simulink model "Ueberholmanoever_david"  (R2018a)
settings: Solver=ode1  StartTime=0.0  StopTime=inf  FixedStep=1/10  RelTol=1e-3  EnableMultiTasking=on
undefined symbols (not defined in the file): finding, gray, Lane, PiCar_library, Rec, SDTV
libraries: simulink x15, visiontextngfix x2, visiontransforms x2, visionconversions x1, visionanalysis x1, visionstatistics x1, embdlinuxlib x1
(part 1 of 2)
settings Model: SimulationMode=external  Creator=raspberry  LastModifiedBy=dave
settings SolverCC: PositivePriorityOrder=on
settings OptimizationCC: PassReuseOutputArgsAs=Individual arguments  MaxStackSize=64
settings DebuggingCC: ParameterTunabilityLossMsg=error
settings HardwareCC: ProdBitPerPointer=32  ProdBitPerSizeT=32  ProdBitPerPtrDiffT=32  ProdLargestAtomicInteger=Long  ProdLargestAtomicFloat=Double  ProdWordSize=32  ProdHWDeviceType=ARM Compatible->ARM Cortex
settings RTWCC: SystemTargetFile=ert.tlc  HardwareBoard=Raspberry Pi  TLCOptions="-aInlineSetEventsForThisBaseRateFcn=TLC_FALSE -aSuppressMultiTaskScheduler=TLC_FALSE  -aRateBasedStepFcn=0"  TemplateMakefile=ert_default_tmf  Toolchain=GNU GCC Raspberry Pi
settings RTWCC: CustomTerminator=|
  | /* Send ALL_LED_OFF Signal to all PWM driver chip address
  | See PCA9685 user manual, section 7.3.4
  | Set Chip in sleep mode, section 7.3.1
  | Reset the PWM ON/OFF states for all LEDs */
  | 
  | int fd;
  | 
  | fd = wiringPiI2CSetup(0x70);
  | wiringPiI2CWriteReg8(fd, 0x00, 0x11); // sleep mode
  | wiringPiI2CWriteReg8(fd, 0xFD, 0x10); // all LED off
  | wiringPiI2CWriteReg8(fd, 0xFC, 0x00);
  | wiringPiI2CWriteReg8(fd, 0xFB, 0x00);
  | wiringPiI2CWriteReg8(fd, 0xFA, 0x00);
settings CodeAppCC: ForceParamTrailComments=on  IgnoreCustomStorageClasses=off  OperatorAnnotations=on  SimulinkDataObjDesc=on  SFDataObjDesc=on  MATLABFcnDesc=on  InsertBlockDesc=on  StateflowObjectComments=on  MATLABSourceComments=on
settings ERTTargetCC: SupportVariableSizeSignals=on  ExtMode=on  ExtModeMexArgs='192.168.43.133' 0 17725

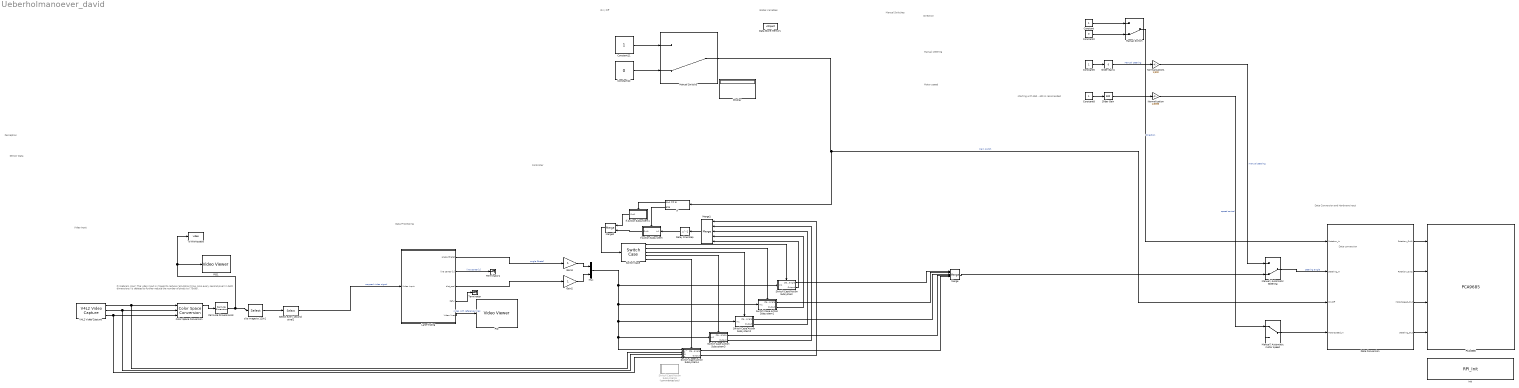
== system Ueberholmanoever_david ==
  note: Manual steering
  note: Sensor Data
  note: Data conversion
  note: Manual Switches
  note: Controller
  note: starting with 350 - 400 is recomended
  note: Data Processing
  note: Data Conversion and Hardware Input
  note: Perception
  note: Pi Webcam Input:
      | The video input is clipped to reduce calculation time. Also every second pixel (in both dimensions) is deleted to further reduce the number of pixels
      | to (75x80).
  note: Direction
  note: Motor speed
  note: Video Input
  note: On / Off
  note: Global Variables
  Color Space Conversion : visionconversions/Color Space  Conversion  conversion=Obsolete  conversionActive=R'G'B' to Y'CbCr  wp_str=D65  rec=Rec. 601 (SDTV)  sys=1125/60/2:1  imagePorts=Separate color signals
      settings: SourceProductName=Computer Vision System Toolbox
  Constant{,5,8,11} (4 alike) : Constant
  Constant12 : Constant  Value=0
  Constant2 : Constant  Value=0
  Data Conversion : Subsystem  AncestorBlock=PiCar_library/Verarbeitung und Datenkonvertierung
  Data Store Memory : DataStoreMemory  DataStoreName=vObject  ReadBeforeWriteMsg=warning  WriteAfterWriteMsg=warning  WriteAfterReadMsg=warning  ShowAdditionalParam=off
  Delay One Step : Delay  DelayLength=1  InitialCondition=1
  Display : Display
  Gain2 : Gain
  Gain3 : Gain
  If : If  IfExpression=u1 == 0
  If Action Subsystem : Subsystem  TreatAsAtomicUnit=on
  If Action Subsystem1 : Subsystem  TreatAsAtomicUnit=on
  Init : S-Function  Priority=1  InitFcn=try, set_param(gcb,'FunctionName','RPI_Init'), end  FunctionName=RPI_Init  SFunctionModules=RPI_Init_wrapper  SFunctionDeploymentMode=off  EnableBusSupport=off  mask(S-Function Builder){}
      mask help: Simulink:masks:SFunctionBuilder_MD
      mask init:
      | val = [[.9  0.75 0.75 1 1 .9 .9 1]',[1 1 0.75 0.75 .9 .9 1 .9]'];try , sys = get_param(gcb,'SfunBuilderFcnName');if isempty(sys), sys = get_param(gcb,'FunctionName'); end,catch, sys = get_param(gcb,'FunctionName'); end
      settings: CopyFcn=set_param(gcbh,'LinkStatus','none')  PreSaveFcn=try, set_param(gcb,'FunctionName','RPI_Init'), end  OpenFcn=sfunctionwizard(gcbh)
      mask Display:
      | plot(val(:,1),val(:,2))
      | disp(sys)
  Lane-finding : Subsystem  AncestorBlock=PiCar_library/Lane-finding
  Manual / Automatic Steering : ManualSwitch  CurrentSetting=0
  "Manual / Automatic motor speed " : ManualSwitch
  Manual Switch : ManualSwitch  CurrentSetting=0
  Manual Switch5 : ManualSwitch  CurrentSetting=0
  Merge : Merge  Inputs=6  InitialOutput=0
  Merge1 : Merge  Inputs=5
  Merge2 : Merge
  Mux : Mux  Inputs=2
  Normalization : Gain  Gain=1/3395
  Normalization1 : Gain  Gain=1/300
  PCA6585 : S-Function  InitFcn=try, set_param(gcb,'FunctionName','PCA9685'), end  FunctionName=PCA9685  SFunctionModules=PCA9685_wrapper  SFunctionDeploymentMode=off  EnableBusSupport=off  mask(S-Function Builder){}
      mask help: Simulink:masks:SFunctionBuilder_MD
      mask init: same as Ueberholmanoever_david/Init
      settings: CopyFcn=set_param(gcbh,'LinkStatus','none')  PreSaveFcn=try, set_param(gcb,'FunctionName','PCA9685'), end  OpenFcn=sfunctionwizard(gcbh)
      mask Display: plot(val(:,1),val(:,2)),disp(sys), port_label('input',1,'IN_1'), port_label('input',2,'IN_2'), port_label('input',3,'PWM'), port_label('input',4,'SERVO')
  PID : VideoViewer  colormapValue=gray(256)  FigPos=[6 1073 939 353]
  PID1 : VideoViewer  colormapValue=gray(256)  FigPos=[1 1038 1539.2 765.6]  OpenAtMdlStart=off
  Permute Dimensions3 : PermuteDimensions
  Select every second pixel2 : Selector  NumberOfDimensions=2  InputPortWidth=3  IndexOptions=Select all,Index vector (dialog)  Indices=[1:2:80],[1:2:160]  OutputSizes=1,1
  Slider Gain : simulink/Math Operations/Slider Gain  gain=500  low=0  high=3395
  Slider Gain1 : simulink/Math Operations/Slider Gain  gain=0  low=-300  high=300
  Switch Case : SwitchCase  CaseConditions={5,4,3,2,1}  ShowDefaultCase=off
  Switch Case Action Subsystem : Subsystem  TreatAsAtomicUnit=on
  Switch Case Action Subsystem1 : Subsystem  TreatAsAtomicUnit=on
  Switch Case Action Subsystem2 : Subsystem  TreatAsAtomicUnit=on
  Switch Case Action Subsystem3 : Subsystem  TreatAsAtomicUnit=on
  Switch Case Action Subsystem4 : Subsystem  TreatAsAtomicUnit=on
  Switch Case Action Subsystem5 : Subsystem  Commented=on  TreatAsAtomicUnit=on
  Terminator : Terminator
  Terminator1 : Terminator
  To Workspace : ToWorkspace  VariableName=video  SaveFormat=Timeseries  SampleTime=-1
  V4L2 Video Capture : embdlinuxlib/V4L2 Video Capture  m_devName='/dev/video0'  roi=[0, 0, 640, 480]  imSizeSelection=320x240  imSize=[640, 480]  pixelFormat=RGB  pixelOrder=Planar  sampleTime=1/10  simOutput=Colorbars  blockPlatform=Raspberry Pi
      settings: SourceProductName=Simulink Support Package for Raspberry Pi Hardware  SourceProductBaseCode=RASPPI
  clip image to 120x1 : Selector  NumberOfDimensions=2  InputPortWidth=3  IndexOptions=Index vector (dialog),Index vector (dialog)  Indices=[150:1:210],[1:2:320]  OutputSizes=1,1
  wires:
  Permute Dimensions3/1 -> clip image to 120x1/1, PID1/1, To Workspace/1
  Color Space Conversion/1 -> Permute Dimensions3/1
  V4L2 Video Capture/3 -> Switch Case Action Subsystem4/4(B), Color Space Conversion/3
  Gain2/1 -> Mux/2
  Lane-finding/5(Video lines) -> PID/1  "video with reference lines"
  Normalization1/1 -> Manual / Automatic Steering/1  "manual steering"
  Constant2/1 -> Manual Switch/2
  Data Conversion/4(Steering_Out) -> PCA6585/4
  Slider Gain/1 -> Normalization/1
  V4L2 Video Capture/1 -> Switch Case Action Subsystem4/2(R), Color Space Conversion/1
  Manual Switch/1 -> Data Conversion/1(Rotation_In)  "Direction"
  Lane-finding/1(angle [theta]) -> Gain3/1  "angle [theta]"
  Normalization/1 -> "Manual / Automatic motor speed "/1  "speed control"
  Select every second pixel2/1 -> Lane-finding/1(Video input)  "cropped video signal"
  Lane-finding/4(Ref_I) -> Terminator/1
  Data Conversion/2(Rotation_Out2) -> PCA6585/2
  Manual / Automatic Steering/1 -> Data Conversion/2(Steering_In)  "steering angle"
  Manual Switch5/1 -> If/1, Data Conversion/3(On/Off)  "main switch"
  Data Conversion/1(Rotation_Out1) -> PCA6585/1
  Data Conversion/3(MotorSpeed_Out) -> PCA6585/3
  Lane-finding/2(line center [y]) -> Terminator1/1  "line center [y]"
  Slider Gain1/1 -> Normalization1/1  "Manual steering"
  Constant5/1 -> Slider Gain1/1
  Constant/1 -> Manual Switch/1
  Constant8/1 -> Slider Gain/1
  Gain3/1 -> Mux/1
  clip image to 120x1/1 -> Select every second pixel2/1
  V4L2 Video Capture/2 -> Switch Case Action Subsystem4/3(G), Color Space Conversion/2
  Constant12/1 -> Manual Switch5/2
  Constant11/1 -> Manual Switch5/1
  "Manual / Automatic motor speed "/1 -> Data Conversion/4(MotorSpeed_In)
  Mux/1 -> Switch Case Action Subsystem4/1(In1), Switch Case Action Subsystem3/1(In2), Switch Case Action Subsystem2/1(In1), Switch Case Action Subsystem1/1(In1), Switch Case Action Subsystem/1(In1)
  Lane-finding/3(dist_real) -> Gain2/1
  Switch Case/1 -> Switch Case Action Subsystem/Action
  Switch Case/2 -> Switch Case Action Subsystem1/Action
  Switch Case/3 -> Switch Case Action Subsystem2/Action
  Switch Case/4 -> Switch Case Action Subsystem3/Action
  Switch Case/5 -> Switch Case Action Subsystem4/Action
  Switch Case Action Subsystem/1(steering angle) -> Merge/1
  Switch Case Action Subsystem1/1(steering angle) -> Merge/2
  Switch Case Action Subsystem2/1(steering angle) -> Merge/3
  Switch Case Action Subsystem3/1(steering angle) -> Merge/4
  Switch Case Action Subsystem4/1(steering angle) -> Merge/5
  Merge/1 -> Manual / Automatic Steering/2
  Switch Case Action Subsystem1/2(Output) -> Merge1/4
  Switch Case Action Subsystem2/2(Output) -> Merge1/3
  Switch Case Action Subsystem3/2(Output) -> Merge1/2
  Switch Case Action Subsystem4/2(Output) -> Merge1/1
  Merge1/1 -> Delay One Step/1
  Switch Case Action Subsystem/2(Output) -> Merge1/5
  If/2 -> If Action Subsystem/Action
  Delay One Step/1 -> If Action Subsystem/1(In1)
  If/1 -> If Action Subsystem1/Action
  If Action Subsystem1/1(Out1) -> Merge2/1
  If Action Subsystem/1(Out1) -> Merge2/2
  Merge2/1 -> Switch Case/1

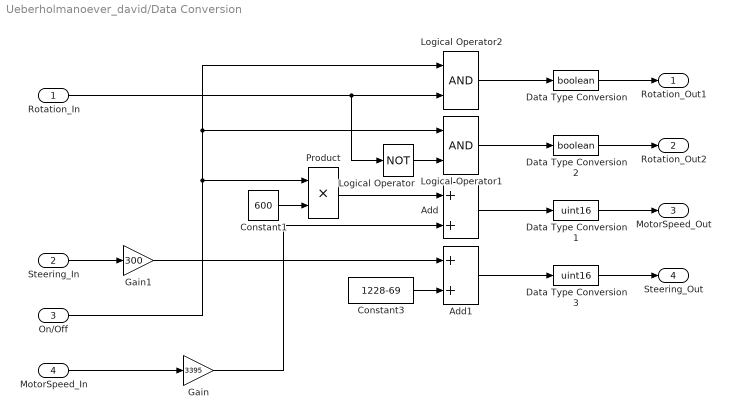
== system Ueberholmanoever_david/Data Conversion ==
  Rotation_In : Inport
  Steering_In : Inport  Port=2
  On/Off : Inport  Port=3
  MotorSpeed_In : Inport  Port=4
  Add : Sum
  Add1 : Sum
  Constant1 : Constant  Value=600
  Constant3 : Constant  Value=1228-69  OutMin=819  OutMax=1638
  Data Type Conversion : DataTypeConversion  OutDataTypeStr=boolean
  Data Type Conversion1 : DataTypeConversion  OutDataTypeStr=uint16
  Data Type Conversion2 : DataTypeConversion  OutDataTypeStr=boolean
  Data Type Conversion3 : DataTypeConversion  OutDataTypeStr=uint16
  Gain : Gain  Gain=3395
  Gain1 : Gain  Gain=300
  Logical Operator : Logic  Operator=NOT  AllPortsSameDT=off  OutDataTypeStr=boolean
  Logical Operator1 : Logic  AllPortsSameDT=off  OutDataTypeStr=boolean
  Logical Operator2 : Logic  AllPortsSameDT=off  OutDataTypeStr=boolean
  Product : Product
  Rotation_Out1 : Outport
  Rotation_Out2 : Outport  Port=2
  MotorSpeed_Out : Outport  Port=3
  Steering_Out : Outport  Port=4
  wires:
  Gain1/1 -> Add1/1
  Gain/1 -> Add/2
  Steering_In/1 -> Gain1/1
  Data Type Conversion/1 -> Rotation_Out1/1
  MotorSpeed_In/1 -> Gain/1
  Data Type Conversion2/1 -> Rotation_Out2/1
  Data Type Conversion3/1 -> Steering_Out/1
  Data Type Conversion1/1 -> MotorSpeed_Out/1
  Product/1 -> Add/1
  Constant1/1 -> Product/2
  Add1/1 -> Data Type Conversion3/1
  Add/1 -> Data Type Conversion1/1
  Rotation_In/1 -> Logical Operator2/2, Logical Operator/1
  Constant3/1 -> Add1/2
  On/Off/1 -> Product/1, Logical Operator2/1, Logical Operator1/1
  Logical Operator/1 -> Logical Operator1/2
  Logical Operator2/1 -> Data Type Conversion/1
  Logical Operator1/1 -> Data Type Conversion2/1

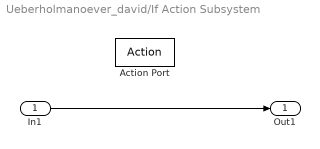
== system Ueberholmanoever_david/If Action Subsystem ==
  In1 : Inport
  Action Port : ActionPort  ActionType=else
  Out1 : Outport
  wires:
  In1/1 -> Out1/1

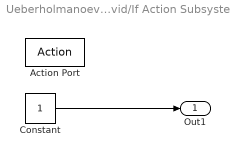
== system Ueberholmanoever_david/If Action Subsystem1 ==
  Action Port : ActionPort  ActionType=then
  Constant : Constant
  Out1 : Outport
  wires:
  Constant/1 -> Out1/1

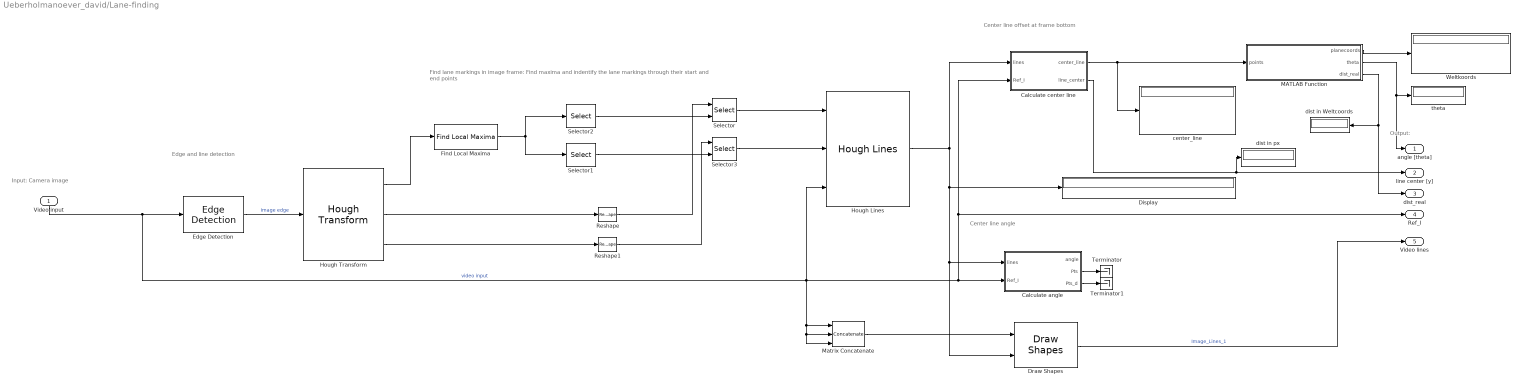
== system Ueberholmanoever_david/Lane-finding ==
  note: Output:
  note: Input: Camera image
  note: Edge and line detection
  note: Find lane markings in image frame:
      | Find maxima and indentify the lane markings through their start and end points
  note: Center line angle
  note: Center line offset at frame bottom
  Video input : Inport
  Calculate angle : MATLAB Function  TreatAsAtomicUnit=on
  Calculate center line : MATLAB Function  TreatAsAtomicUnit=on
  Display : Display
  Draw Shapes : visiontextngfix/Draw Shapes  shape=Lines  fill=off  lineWidth=1  fillClrSource=Specify via dialog  display=User-specified value  intensity=200  color=[0 0 255]  opacity=0.6  viewport=Entire image  antialiasing=off  inType=Obsolete  imagePorts=One multidimensional signal  prodOutputMode=Binary point scaling  prodOutputWordLength=32  prodOutputFracLength=14  memoryMode=Specify word length  memoryWordLength=16  memoryFracLength=14  roundingMode=Floor  overflowMode=off
      settings: SourceProductName=Computer Vision System Toolbox
  Edge Detection : visionanalysis/Edge Detection  method=Sobel  outputType=Binary image  userDefinedThreshold=off  thresholdSource=Input port  threshold=20  thresholdTuning=4  edgeThinning=off  threshold_canny=[0.25 0.60]  autoPercent=70  sigma=1  roundingMode=Floor  overflowMode=off  prodOutputMode=Binary point scaling  prodOutputWordLength=32  prodOutputFracLength=8  prodOutputSlope=2^-8  accumSlope=2^-8  outputSlope=2^-4
      settings: SourceProductName=Computer Vision System Toolbox  SourceProductBaseCode=VP
  Find Local Maxima : visionstatistics/Find Local Maxima  num_peaks=2  nhood_size=[5 7]  src_thresh=Obsolete9b  src_thresh_inuse=Specify via dialog  threshold=10  inputIsHough=off  dt_peak=uint32  isOutVarDim=on  dt_count=uint32
      settings: SourceProductName=Computer Vision System Toolbox  SourceProductBaseCode=VP
  Hough Lines : visiontransforms/Hough Lines  sineCompMethod=Trigonometric function  thetaRes=pi/180  firstCoeffMode=Specify word length  firstCoeffWordLength=16  firstCoeffFracLength=15  prodOutputMode=Binary point scaling  prodOutputWordLength=32  prodOutputFracLength=16  roundingMode=Nearest  overflowMode=on
      settings: SourceProductName=Computer Vision System Toolbox  SourceProductBaseCode=VP
  Hough Transform : visiontransforms/Hough Transform  theta_res=pi/180  rho_res=1  out_theta_rho=on  outdtmode=double  firstCoeffMode=Binary point scaling  firstCoeffWordLength=16  firstCoeffFracLength=14  secondCoeffMode=Binary point scaling  secondCoeffWordLength=32  secondCoeffFracLength=16  outputMode=Binary point scaling  outputWordLength=16  outputFracLength=0  accumMode=Binary point scaling  accumWordLength=32  accumFracLength=20  prodOutputMode=Binary point scaling  prodOutputWordLength=32  prodOutputFracLength=20  memoryMode=Binary point scaling  memoryWordLength=32  memoryFracLength=16  roundingMode=Nearest  overflowMode=on
      settings: SourceProductName=Computer Vision System Toolbox  SourceProductBaseCode=VP
  MATLAB Function : MATLAB Function  TreatAsAtomicUnit=on
  Matrix Concatenate : Concatenate  NumInputs=3  Mode=Multidimensional array  ConcatenateDimension=3
  Reshape : Reshape
  Reshape1 : Reshape
  Selector : Selector  IndexOptions=Index vector (port)  Indices=[1 3]  OutputSizes=1
  Selector1 : Selector  NumberOfDimensions=2  InputPortWidth=3  IndexOptions=Select all,Index vector (dialog)  Indices=[1 3],2  OutputSizes=1,1
  Selector2 : Selector  NumberOfDimensions=2  InputPortWidth=3  IndexOptions=Select all,Index vector (dialog)  Indices=[1 3],1  OutputSizes=1,1
  Selector3 : Selector  IndexOptions=Index vector (port)  Indices=[1 3]  OutputSizes=1
  Terminator : Terminator
  Terminator1 : Terminator
  Weltkoords : Display
  center_line : Display
  dist in Weltcoords : Display
  dist in px : Display
  theta : Display
  angle [theta] : Outport
  line center [y] : Outport  Port=2
  dist_real : Outport  Port=3
  Ref_I : Outport  Port=4
  Video lines : Outport  Port=5
  wires:
  Calculate center line/2(line_center) -> dist in px/1, line center [y]/1
  Hough Lines/1 -> Calculate angle/1(lines), Draw Shapes/2, Display/1, Calculate center line/1(lines)
  Draw Shapes/1 -> Video lines/1  "Image_Lines_1"
  Matrix Concatenate/1 -> Draw Shapes/1
  Reshape1/1 -> Selector3/1
  Selector3/1 -> Hough Lines/2
  Reshape/1 -> Selector/1
  Selector/1 -> Hough Lines/1
  Find Local Maxima/1 -> Selector1/1, Selector2/1
  Selector2/1 -> Selector/2
  Selector1/1 -> Selector3/2
  Hough Transform/1 -> Find Local Maxima/1
  Hough Transform/3 -> Reshape1/1
  Hough Transform/2 -> Reshape/1
  Video input/1 -> Edge Detection/1, Matrix Concatenate/3, Matrix Concatenate/2, Matrix Concatenate/1, Hough Lines/3, Ref_I/1, Calculate center line/2(Ref_I), Calculate angle/2(Ref_I)  "video input"
  Edge Detection/1 -> Hough Transform/1  "Image edge"
  Calculate angle/3(Pts_d) -> Terminator1/1
  Calculate angle/2(Pts) -> Terminator/1
  MATLAB Function/1(planecoords) -> Weltkoords/1
  MATLAB Function/2(theta) -> angle [theta]/1, theta/1
  Calculate center line/1(center_line) -> MATLAB Function/1(points), center_line/1
  MATLAB Function/3(dist_real) -> dist in Weltcoords/1, dist_real/1

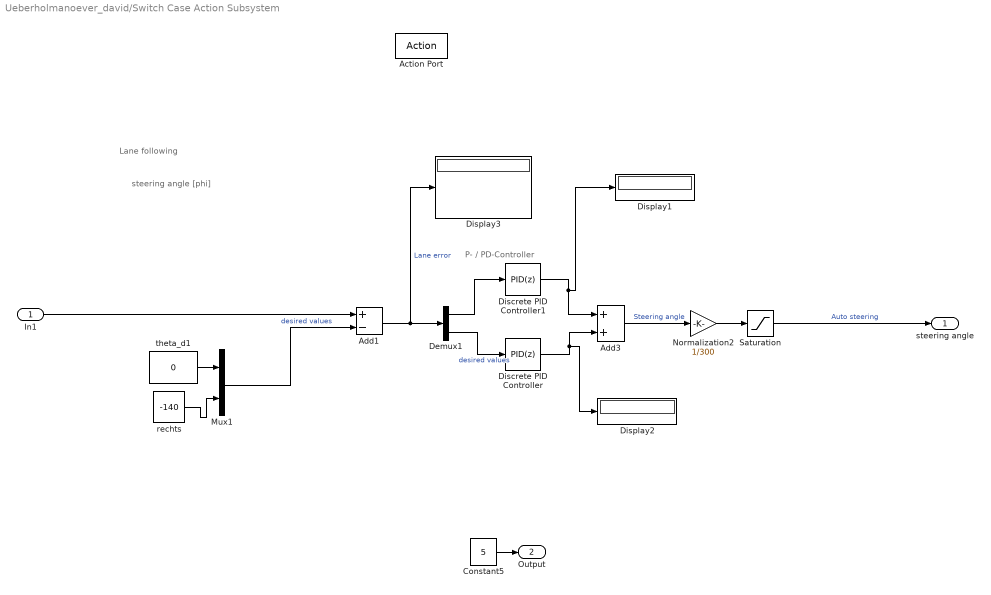
== system Ueberholmanoever_david/Switch Case Action Subsystem ==
  note: steering angle [phi]
  note: P- / PD-Controller
  note: Lane following
  In1 : Inport
  Action Port : ActionPort  ActionType=case
  Add1 : Sum  Inputs=+-
  Add3 : Sum
  Constant5 : Constant  Value=5  OutDataTypeStr=uint8
  Demux1 : Demux  Outputs=2
  Discrete PID Controller : simulink/Continuous/PID Controller  Controller=PID  TimeDomain=Discrete-time  SampleTime=-1  IntegratorMethod=Forward Euler  FilterMethod=Forward Euler  Form=Parallel  UseFilter=on  ControllerParametersSource=internal  P=0.2  I=0  D=0  N=100  InitialConditionSource=internal  InitialConditionForIntegrator=0  InitialConditionForFilter=0  ExternalReset=none  LimitOutput=off  UpperSaturationLimit=inf  LowerSaturationLimit=-inf  LinearizeAsGain=off  AntiWindupMode=none  Kb=1  TrackingMode=off  Kt=1  PParamMin=[]  PParamMax=[]  IParamMin=[]  IParamMax=[]  DParamMin=[]  DParamMax=[]  NParamMin=[]  NParamMax=[]  KbParamMin=[]  KbParamMax=[]  KtParamMin=[]  KtParamMax=[]  POutMin=[]  POutMax=[]  IOutMin=[]  IOutMax=[]  DOutMin=[]  DOutMax=[]  NOutMin=[]  NOutMax=[]  KbOutMin=[]  KbOutMax=[]  KtOutMin=[]  KtOutMax=[]  IntegratorOutMin=[]  IntegratorOutMax=[]  FilterOutMin=[]  FilterOutMax=[]  SumOutMin=[]  SumOutMax=[]  SumI1OutMin=[]  SumI1OutMax=[]  SumI2OutMin=[]  SumI2OutMax=[]  SumI3OutMin=[]  SumI3OutMax=[]  SumDOutMin=[]  SumDOutMax=[]  SaturationOutMin=[]  SaturationOutMax=[]  IntegratorContinuousStateAttributes=''  IntegratorStateMustResolveToSignalObject=off  IntegratorRTWStateStorageClass=Auto  FilterContinuousStateAttributes=''  FilterStateMustResolveToSignalObject=off  FilterRTWStateStorageClass=Auto  DifferentiatorICPrevScaledInput=0  DifferentiatorOutMin=[]  DifferentiatorOutMax=[]  FilterDiffOutCoefMin=[]  FilterDiffOutCoefMax=[]  SumDenOutMin=[]  SumDenOutMax=[]  SumNumOutMin=[]  SumNumOutMax=[]  ReciprocalOutMin=[]  ReciprocalOutMax=[]  DivideOutMin=[]  DivideOutMax=[]  TunerSelectOption=Transfer Function Based (PID Tuner App)
  Discrete PID Controller1 : simulink/Continuous/PID Controller  Controller=PID  TimeDomain=Discrete-time  SampleTime=-1  IntegratorMethod=Forward Euler  FilterMethod=Forward Euler  Form=Parallel  UseFilter=on  ControllerParametersSource=internal  P=6  I=0  D=0  N=100  InitialConditionSource=internal  InitialConditionForIntegrator=0  InitialConditionForFilter=0  ExternalReset=none  LimitOutput=off  UpperSaturationLimit=inf  LowerSaturationLimit=-inf  LinearizeAsGain=off  AntiWindupMode=none  Kb=1  TrackingMode=off  Kt=1  PParamMin=[]  PParamMax=[]  IParamMin=[]  IParamMax=[]  DParamMin=[]  DParamMax=[]  NParamMin=[]  NParamMax=[]  KbParamMin=[]  KbParamMax=[]  KtParamMin=[]  KtParamMax=[]  POutMin=[]  POutMax=[]  IOutMin=[]  IOutMax=[]  DOutMin=[]  DOutMax=[]  NOutMin=[]  NOutMax=[]  KbOutMin=[]  KbOutMax=[]  KtOutMin=[]  KtOutMax=[]  IntegratorOutMin=[]  IntegratorOutMax=[]  FilterOutMin=[]  FilterOutMax=[]  SumOutMin=[]  SumOutMax=[]  SumI1OutMin=[]  SumI1OutMax=[]  SumI2OutMin=[]  SumI2OutMax=[]  SumI3OutMin=[]  SumI3OutMax=[]  SumDOutMin=[]  SumDOutMax=[]  SaturationOutMin=[]  SaturationOutMax=[]  IntegratorContinuousStateAttributes=''  IntegratorStateMustResolveToSignalObject=off  IntegratorRTWStateStorageClass=Auto  FilterContinuousStateAttributes=''  FilterStateMustResolveToSignalObject=off  FilterRTWStateStorageClass=Auto  DifferentiatorICPrevScaledInput=0  DifferentiatorOutMin=[]  DifferentiatorOutMax=[]  FilterDiffOutCoefMin=[]  FilterDiffOutCoefMax=[]  SumDenOutMin=[]  SumDenOutMax=[]  SumNumOutMin=[]  SumNumOutMax=[]  ReciprocalOutMin=[]  ReciprocalOutMax=[]  DivideOutMin=[]  DivideOutMax=[]  TunerSelectOption=Transfer Function Based (PID Tuner App)
  Display1 : Display
  Display2 : Display
  Display3 : Display
  Mux1 : Mux  Inputs=2
  Normalization2 : Gain  Gain=1/300
  Saturation : Saturate  UpperLimit=1  LowerLimit=-1
  rechts : Constant  Value=-140
  theta_d1 : Constant  Value=0
  steering angle : Outport  InitialOutput=[0]
  Output : Outport  Port=2
  wires:
  rechts/1 -> Mux1/2
  Add1/1 -> Display3/1, Demux1/1  "Lane error"
  In1/1 -> Add1/1
  theta_d1/1 -> Mux1/1
  Discrete PID Controller/1 -> Display2/1, Add3/2
  Saturation/1 -> steering angle/1  "Auto steering"
  Normalization2/1 -> Saturation/1
  Discrete PID Controller1/1 -> Display1/1, Add3/1
  Demux1/2 -> Discrete PID Controller/1  "desired values"
  Demux1/1 -> Discrete PID Controller1/1
  Add3/1 -> Normalization2/1  "Steering angle"
  Mux1/1 -> Add1/2  "desired values"
  Constant5/1 -> Output/1

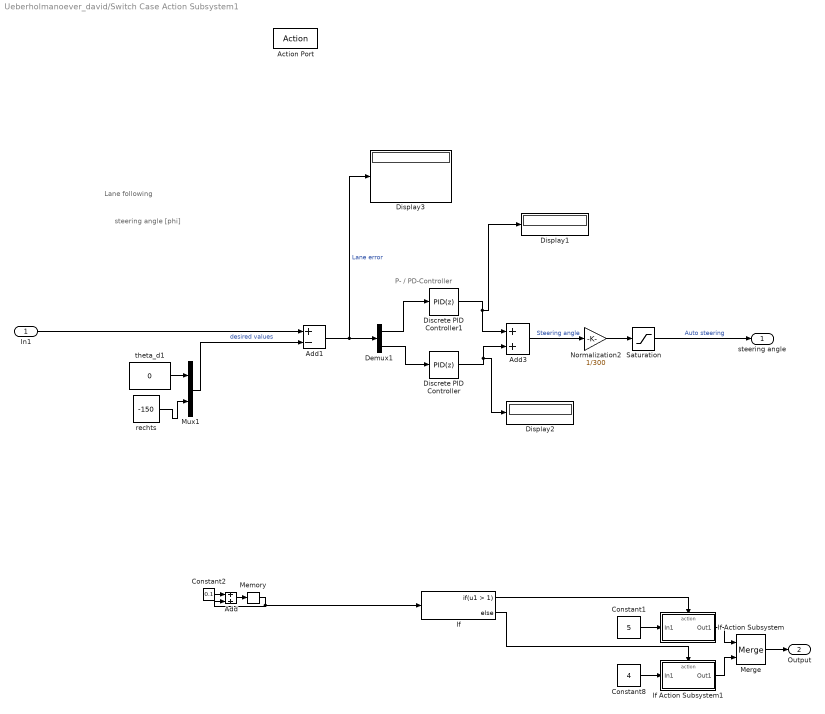
== system Ueberholmanoever_david/Switch Case Action Subsystem1 ==
  note: Lane following
  note: steering angle [phi]
  note: P- / PD-Controller
  In1 : Inport
  Action Port : ActionPort  ActionType=case
  Add : Sum
  Add1 : Sum  Inputs=+-
  Add3 : Sum
  Constant1 : Constant  Value=5  OutDataTypeStr=uint8
  Constant2 : Constant  Value=0.1
  Constant8 : Constant  Value=4  OutDataTypeStr=uint8
  Demux1 : Demux  Outputs=2
  Discrete PID Controller : simulink/Continuous/PID Controller  Controller=PID  TimeDomain=Discrete-time  SampleTime=-1  IntegratorMethod=Forward Euler  FilterMethod=Forward Euler  Form=Parallel  UseFilter=on  ControllerParametersSource=internal  P=0.2  I=0  D=0  N=100  InitialConditionSource=internal  InitialConditionForIntegrator=0  InitialConditionForFilter=0  ExternalReset=none  LimitOutput=off  UpperSaturationLimit=inf  LowerSaturationLimit=-inf  LinearizeAsGain=off  AntiWindupMode=none  Kb=1  TrackingMode=off  Kt=1  PParamMin=[]  PParamMax=[]  IParamMin=[]  IParamMax=[]  DParamMin=[]  DParamMax=[]  NParamMin=[]  NParamMax=[]  KbParamMin=[]  KbParamMax=[]  KtParamMin=[]  KtParamMax=[]  POutMin=[]  POutMax=[]  IOutMin=[]  IOutMax=[]  DOutMin=[]  DOutMax=[]  NOutMin=[]  NOutMax=[]  KbOutMin=[]  KbOutMax=[]  KtOutMin=[]  KtOutMax=[]  IntegratorOutMin=[]  IntegratorOutMax=[]  FilterOutMin=[]  FilterOutMax=[]  SumOutMin=[]  SumOutMax=[]  SumI1OutMin=[]  SumI1OutMax=[]  SumI2OutMin=[]  SumI2OutMax=[]  SumI3OutMin=[]  SumI3OutMax=[]  SumDOutMin=[]  SumDOutMax=[]  SaturationOutMin=[]  SaturationOutMax=[]  IntegratorContinuousStateAttributes=''  IntegratorStateMustResolveToSignalObject=off  IntegratorRTWStateStorageClass=Auto  FilterContinuousStateAttributes=''  FilterStateMustResolveToSignalObject=off  FilterRTWStateStorageClass=Auto  DifferentiatorICPrevScaledInput=0  DifferentiatorOutMin=[]  DifferentiatorOutMax=[]  FilterDiffOutCoefMin=[]  FilterDiffOutCoefMax=[]  SumDenOutMin=[]  SumDenOutMax=[]  SumNumOutMin=[]  SumNumOutMax=[]  ReciprocalOutMin=[]  ReciprocalOutMax=[]  DivideOutMin=[]  DivideOutMax=[]  TunerSelectOption=Transfer Function Based (PID Tuner App)
  Discrete PID Controller1 : simulink/Continuous/PID Controller  Controller=PID  TimeDomain=Discrete-time  SampleTime=-1  IntegratorMethod=Forward Euler  FilterMethod=Forward Euler  Form=Parallel  UseFilter=on  ControllerParametersSource=internal  P=6  I=0  D=0  N=100  InitialConditionSource=internal  InitialConditionForIntegrator=0  InitialConditionForFilter=0  ExternalReset=none  LimitOutput=off  UpperSaturationLimit=inf  LowerSaturationLimit=-inf  LinearizeAsGain=off  AntiWindupMode=none  Kb=1  TrackingMode=off  Kt=1  PParamMin=[]  PParamMax=[]  IParamMin=[]  IParamMax=[]  DParamMin=[]  DParamMax=[]  NParamMin=[]  NParamMax=[]  KbParamMin=[]  KbParamMax=[]  KtParamMin=[]  KtParamMax=[]  POutMin=[]  POutMax=[]  IOutMin=[]  IOutMax=[]  DOutMin=[]  DOutMax=[]  NOutMin=[]  NOutMax=[]  KbOutMin=[]  KbOutMax=[]  KtOutMin=[]  KtOutMax=[]  IntegratorOutMin=[]  IntegratorOutMax=[]  FilterOutMin=[]  FilterOutMax=[]  SumOutMin=[]  SumOutMax=[]  SumI1OutMin=[]  SumI1OutMax=[]  SumI2OutMin=[]  SumI2OutMax=[]  SumI3OutMin=[]  SumI3OutMax=[]  SumDOutMin=[]  SumDOutMax=[]  SaturationOutMin=[]  SaturationOutMax=[]  IntegratorContinuousStateAttributes=''  IntegratorStateMustResolveToSignalObject=off  IntegratorRTWStateStorageClass=Auto  FilterContinuousStateAttributes=''  FilterStateMustResolveToSignalObject=off  FilterRTWStateStorageClass=Auto  DifferentiatorICPrevScaledInput=0  DifferentiatorOutMin=[]  DifferentiatorOutMax=[]  FilterDiffOutCoefMin=[]  FilterDiffOutCoefMax=[]  SumDenOutMin=[]  SumDenOutMax=[]  SumNumOutMin=[]  SumNumOutMax=[]  ReciprocalOutMin=[]  ReciprocalOutMax=[]  DivideOutMin=[]  DivideOutMax=[]  TunerSelectOption=Transfer Function Based (PID Tuner App)
  Display1 : Display
  Display2 : Display
  Display3 : Display
  If : If  IfExpression=u1 > 1
  If Action Subsystem : Subsystem  TreatAsAtomicUnit=on
  If Action Subsystem1 : Subsystem  TreatAsAtomicUnit=on
  Memory : Memory
  Merge : Merge
  Mux1 : Mux  Inputs=2
  Normalization2 : Gain  Gain=1/300
  Saturation : Saturate  UpperLimit=1  LowerLimit=-1
  rechts : Constant  Value=-150
  theta_d1 : Constant  Value=0
  steering angle : Outport  InitialOutput=[0]
  Output : Outport  Port=2
  wires:
  Add3/1 -> Normalization2/1  "Steering angle"
  Saturation/1 -> steering angle/1  "Auto steering"
  Normalization2/1 -> Saturation/1
  Demux1/1 -> Discrete PID Controller1/1
  Discrete PID Controller/1 -> Display2/1, Add3/2
  theta_d1/1 -> Mux1/1
  Discrete PID Controller1/1 -> Display1/1, Add3/1
  Mux1/1 -> Add1/2  "desired values"
  In1/1 -> Add1/1
  Add/1 -> Memory/1
  rechts/1 -> Mux1/2
  Constant2/1 -> Add/1
  Add1/1 -> Display3/1, Demux1/1  "Lane error"
  Demux1/2 -> Discrete PID Controller/1
  Memory/1 -> If/1, Add/2
  If/2 -> If Action Subsystem1/Action
  If/1 -> If Action Subsystem/Action
  Merge/1 -> Output/1
  Constant1/1 -> If Action Subsystem/1(In1)
  Constant8/1 -> If Action Subsystem1/1(In1)
  If Action Subsystem1/1(Out1) -> Merge/2
  If Action Subsystem/1(Out1) -> Merge/1

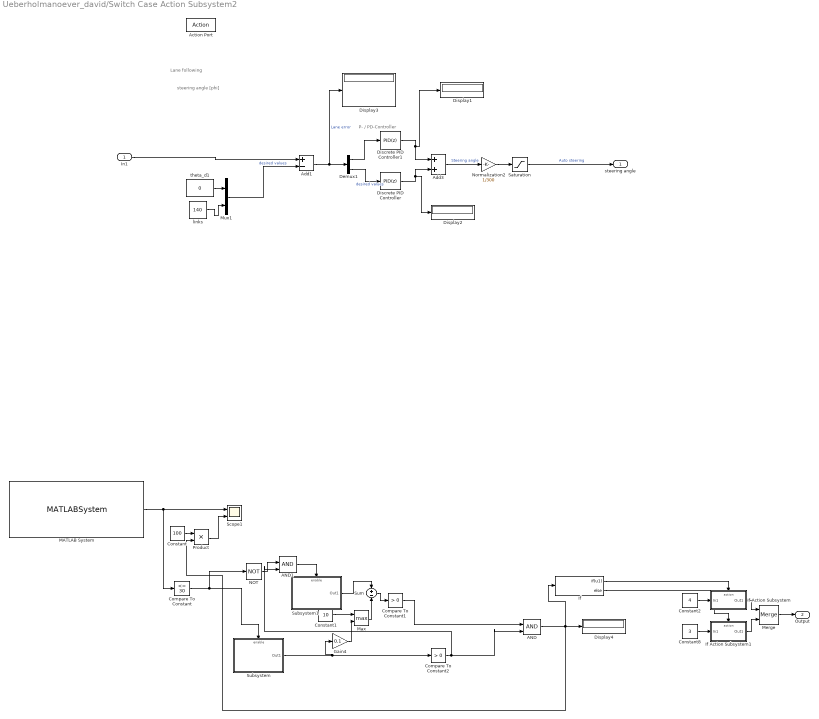
== system Ueberholmanoever_david/Switch Case Action Subsystem2 ==
  note: steering angle [phi]
  note: P- / PD-Controller
  note: Lane following
  In1 : Inport
  Action Port : ActionPort  ActionType=case
  AND : Logic  IconShape=distinctive  AllPortsSameDT=off  OutDataTypeStr=boolean
  AND1 : Logic  IconShape=distinctive  AllPortsSameDT=off  OutDataTypeStr=boolean
  Add1 : Sum  Inputs=+-
  Add3 : Sum
  Compare To Constant : simulink/Logic and Bit Operations/Compare To Constant  relop=<=  const=30  OutDataTypeStr=boolean
  Compare To Constant1 : simulink/Logic and Bit Operations/Compare To Constant  relop=>  const=0  OutDataTypeStr=boolean
  Compare To Constant2 : simulink/Logic and Bit Operations/Compare To Constant  relop=>  const=0  OutDataTypeStr=boolean
  Constant : Constant  Value=100
  Constant1 : Constant  Value=10
  Constant2 : Constant  Value=4  OutDataTypeStr=uint8
  Constant8 : Constant  Value=3  OutDataTypeStr=uint8
  Demux1 : Demux  Outputs=2
  Discrete PID Controller : simulink/Continuous/PID Controller  Controller=PID  TimeDomain=Discrete-time  SampleTime=-1  IntegratorMethod=Forward Euler  FilterMethod=Forward Euler  Form=Parallel  UseFilter=on  ControllerParametersSource=internal  P=0.2  I=0  D=0  N=100  InitialConditionSource=internal  InitialConditionForIntegrator=0  InitialConditionForFilter=0  ExternalReset=none  LimitOutput=off  UpperSaturationLimit=inf  LowerSaturationLimit=-inf  LinearizeAsGain=off  AntiWindupMode=none  Kb=1  TrackingMode=off  Kt=1  PParamMin=[]  PParamMax=[]  IParamMin=[]  IParamMax=[]  DParamMin=[]  DParamMax=[]  NParamMin=[]  NParamMax=[]  KbParamMin=[]  KbParamMax=[]  KtParamMin=[]  KtParamMax=[]  POutMin=[]  POutMax=[]  IOutMin=[]  IOutMax=[]  DOutMin=[]  DOutMax=[]  NOutMin=[]  NOutMax=[]  KbOutMin=[]  KbOutMax=[]  KtOutMin=[]  KtOutMax=[]  IntegratorOutMin=[]  IntegratorOutMax=[]  FilterOutMin=[]  FilterOutMax=[]  SumOutMin=[]  SumOutMax=[]  SumI1OutMin=[]  SumI1OutMax=[]  SumI2OutMin=[]  SumI2OutMax=[]  SumI3OutMin=[]  SumI3OutMax=[]  SumDOutMin=[]  SumDOutMax=[]  SaturationOutMin=[]  SaturationOutMax=[]  IntegratorContinuousStateAttributes=''  IntegratorStateMustResolveToSignalObject=off  IntegratorRTWStateStorageClass=Auto  FilterContinuousStateAttributes=''  FilterStateMustResolveToSignalObject=off  FilterRTWStateStorageClass=Auto  DifferentiatorICPrevScaledInput=0  DifferentiatorOutMin=[]  DifferentiatorOutMax=[]  FilterDiffOutCoefMin=[]  FilterDiffOutCoefMax=[]  SumDenOutMin=[]  SumDenOutMax=[]  SumNumOutMin=[]  SumNumOutMax=[]  ReciprocalOutMin=[]  ReciprocalOutMax=[]  DivideOutMin=[]  DivideOutMax=[]  TunerSelectOption=Transfer Function Based (PID Tuner App)
  Discrete PID Controller1 : simulink/Continuous/PID Controller  Controller=PID  TimeDomain=Discrete-time  SampleTime=-1  IntegratorMethod=Forward Euler  FilterMethod=Forward Euler  Form=Parallel  UseFilter=on  ControllerParametersSource=internal  P=6  I=0  D=0  N=100  InitialConditionSource=internal  InitialConditionForIntegrator=0  InitialConditionForFilter=0  ExternalReset=none  LimitOutput=off  UpperSaturationLimit=inf  LowerSaturationLimit=-inf  LinearizeAsGain=off  AntiWindupMode=none  Kb=1  TrackingMode=off  Kt=1  PParamMin=[]  PParamMax=[]  IParamMin=[]  IParamMax=[]  DParamMin=[]  DParamMax=[]  NParamMin=[]  NParamMax=[]  KbParamMin=[]  KbParamMax=[]  KtParamMin=[]  KtParamMax=[]  POutMin=[]  POutMax=[]  IOutMin=[]  IOutMax=[]  DOutMin=[]  DOutMax=[]  NOutMin=[]  NOutMax=[]  KbOutMin=[]  KbOutMax=[]  KtOutMin=[]  KtOutMax=[]  IntegratorOutMin=[]  IntegratorOutMax=[]  FilterOutMin=[]  FilterOutMax=[]  SumOutMin=[]  SumOutMax=[]  SumI1OutMin=[]  SumI1OutMax=[]  SumI2OutMin=[]  SumI2OutMax=[]  SumI3OutMin=[]  SumI3OutMax=[]  SumDOutMin=[]  SumDOutMax=[]  SaturationOutMin=[]  SaturationOutMax=[]  IntegratorContinuousStateAttributes=''  IntegratorStateMustResolveToSignalObject=off  IntegratorRTWStateStorageClass=Auto  FilterContinuousStateAttributes=''  FilterStateMustResolveToSignalObject=off  FilterRTWStateStorageClass=Auto  DifferentiatorICPrevScaledInput=0  DifferentiatorOutMin=[]  DifferentiatorOutMax=[]  FilterDiffOutCoefMin=[]  FilterDiffOutCoefMax=[]  SumDenOutMin=[]  SumDenOutMax=[]  SumNumOutMin=[]  SumNumOutMax=[]  ReciprocalOutMin=[]  ReciprocalOutMax=[]  DivideOutMin=[]  DivideOutMax=[]  TunerSelectOption=Transfer Function Based (PID Tuner App)
  Display{1..4} (4 alike) : Display
  Gain4 : Gain  Gain=0.1
  If : If  IfExpression=u1
  If Action Subsystem : Subsystem  TreatAsAtomicUnit=on
  If Action Subsystem1 : Subsystem  TreatAsAtomicUnit=on
  MATLAB System : MATLABSystem  System=HCSR04
      mask Type: HCSR04
      mask Display:
      | disp('HC-SR04');
      | port_label('output',1,'distance_cm');
  Max : MinMax  Function=max  Inputs=2
  Merge : Merge
  Mux1 : Mux  Inputs=2
  NOT : Logic  Operator=NOT  IconShape=distinctive  AllPortsSameDT=off  OutDataTypeStr=boolean
  Normalization2 : Gain  Gain=1/300
  Product : Product
  Saturation : Saturate  UpperLimit=1  LowerLimit=-1
  Scope1 : Scope  NumInputPorts=2
  Subsystem : Subsystem
  Subsystem1 : Subsystem
  Sum : Sum  Inputs=+-
  links : Constant  Value=140
  theta_d1 : Constant  Value=0
  steering angle : Outport  InitialOutput=[0]
  Output : Outport  Port=2
  wires:
  Discrete PID Controller1/1 -> Display1/1, Add3/1
  Compare To Constant/1 -> Subsystem/Enable, NOT/1
  links/1 -> Mux1/2
  Mux1/1 -> Add1/2  "desired values"
  Normalization2/1 -> Saturation/1
  Constant1/1 -> Max/1
  AND1/1 -> Subsystem1/Enable
  NOT/1 -> AND1/1
  Demux1/2 -> Discrete PID Controller/1  "desired values"
  Add1/1 -> Display3/1, Demux1/1  "Lane error"
  MATLAB System/1 -> Compare To Constant/1, Scope1/1
  theta_d1/1 -> Mux1/1
  Constant/1 -> Product/1
  Sum/1 -> Compare To Constant1/1
  Compare To Constant2/1 -> AND1/2, AND/2
  Discrete PID Controller/1 -> Display2/1, Add3/2
  AND/1 -> If/1, Product/2, Display4/1
  Product/1 -> Scope1/2
  Add3/1 -> Normalization2/1  "Steering angle"
  Saturation/1 -> steering angle/1  "Auto steering"
  Subsystem/1(Out1) -> Gain4/1, Compare To Constant2/1
  In1/1 -> Add1/1
  Compare To Constant1/1 -> AND/1
  Subsystem1/1(Out1) -> Sum/1
  Max/1 -> Sum/2
  Demux1/1 -> Discrete PID Controller1/1
  Gain4/1 -> Max/2
  If/2 -> If Action Subsystem1/Action
  Merge/1 -> Output/1
  Constant8/1 -> If Action Subsystem1/1(In1)
  If Action Subsystem1/1(Out1) -> Merge/2
  If Action Subsystem/1(Out1) -> Merge/1
  If/1 -> If Action Subsystem/Action
  Constant2/1 -> If Action Subsystem/1(In1)

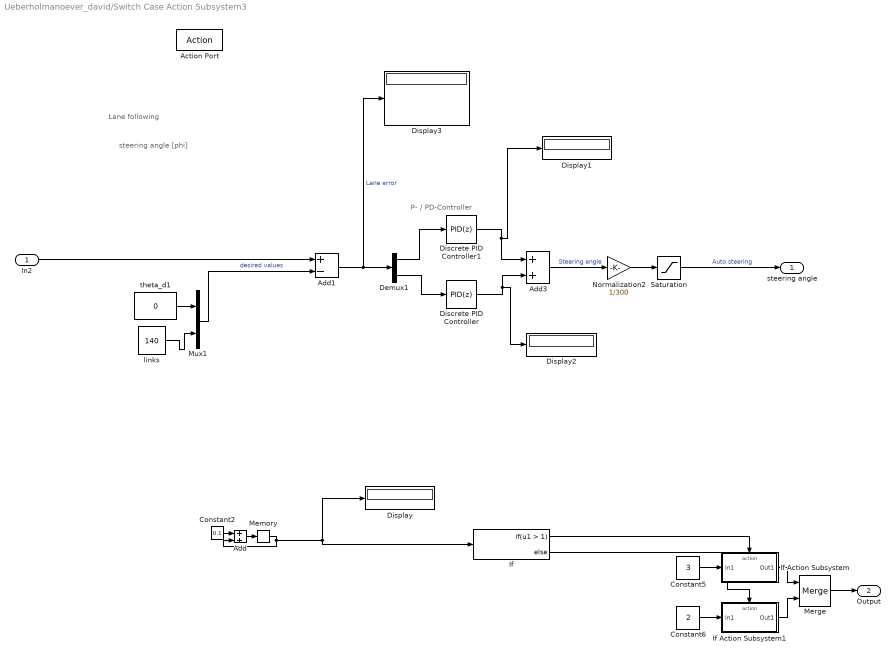
== system Ueberholmanoever_david/Switch Case Action Subsystem3 ==
  note: Lane following
  note: P- / PD-Controller
  note: steering angle [phi]
  In2 : Inport
  Action Port : ActionPort  ActionType=case
  Add : Sum
  Add1 : Sum  Inputs=+-
  Add3 : Sum
  Constant2 : Constant  Value=0.1
  Constant5 : Constant  Value=3  OutDataTypeStr=uint8
  Constant6 : Constant  Value=2  OutDataTypeStr=uint8
  Demux1 : Demux  Outputs=2
  Discrete PID Controller : simulink/Continuous/PID Controller  Controller=PID  TimeDomain=Discrete-time  SampleTime=-1  IntegratorMethod=Forward Euler  FilterMethod=Forward Euler  Form=Parallel  UseFilter=on  ControllerParametersSource=internal  P=0.4  I=0  D=0  N=100  InitialConditionSource=internal  InitialConditionForIntegrator=0  InitialConditionForFilter=0  ExternalReset=none  LimitOutput=off  UpperSaturationLimit=inf  LowerSaturationLimit=-inf  LinearizeAsGain=off  AntiWindupMode=none  Kb=1  TrackingMode=off  Kt=1  PParamMin=[]  PParamMax=[]  IParamMin=[]  IParamMax=[]  DParamMin=[]  DParamMax=[]  NParamMin=[]  NParamMax=[]  KbParamMin=[]  KbParamMax=[]  KtParamMin=[]  KtParamMax=[]  POutMin=[]  POutMax=[]  IOutMin=[]  IOutMax=[]  DOutMin=[]  DOutMax=[]  NOutMin=[]  NOutMax=[]  KbOutMin=[]  KbOutMax=[]  KtOutMin=[]  KtOutMax=[]  IntegratorOutMin=[]  IntegratorOutMax=[]  FilterOutMin=[]  FilterOutMax=[]  SumOutMin=[]  SumOutMax=[]  SumI1OutMin=[]  SumI1OutMax=[]  SumI2OutMin=[]  SumI2OutMax=[]  SumI3OutMin=[]  SumI3OutMax=[]  SumDOutMin=[]  SumDOutMax=[]  SaturationOutMin=[]  SaturationOutMax=[]  IntegratorContinuousStateAttributes=''  IntegratorStateMustResolveToSignalObject=off  IntegratorRTWStateStorageClass=Auto  FilterContinuousStateAttributes=''  FilterStateMustResolveToSignalObject=off  FilterRTWStateStorageClass=Auto  DifferentiatorICPrevScaledInput=0  DifferentiatorOutMin=[]  DifferentiatorOutMax=[]  FilterDiffOutCoefMin=[]  FilterDiffOutCoefMax=[]  SumDenOutMin=[]  SumDenOutMax=[]  SumNumOutMin=[]  SumNumOutMax=[]  ReciprocalOutMin=[]  ReciprocalOutMax=[]  DivideOutMin=[]  DivideOutMax=[]  TunerSelectOption=Transfer Function Based (PID Tuner App)
  Discrete PID Controller1 : simulink/Continuous/PID Controller  Controller=PID  TimeDomain=Discrete-time  SampleTime=-1  IntegratorMethod=Forward Euler  FilterMethod=Forward Euler  Form=Parallel  UseFilter=on  ControllerParametersSource=internal  P=10  I=0  D=0  N=100  InitialConditionSource=internal  InitialConditionForIntegrator=0  InitialConditionForFilter=0  ExternalReset=none  LimitOutput=off  UpperSaturationLimit=inf  LowerSaturationLimit=-inf  LinearizeAsGain=off  AntiWindupMode=none  Kb=1  TrackingMode=off  Kt=1  PParamMin=[]  PParamMax=[]  IParamMin=[]  IParamMax=[]  DParamMin=[]  DParamMax=[]  NParamMin=[]  NParamMax=[]  KbParamMin=[]  KbParamMax=[]  KtParamMin=[]  KtParamMax=[]  POutMin=[]  POutMax=[]  IOutMin=[]  IOutMax=[]  DOutMin=[]  DOutMax=[]  NOutMin=[]  NOutMax=[]  KbOutMin=[]  KbOutMax=[]  KtOutMin=[]  KtOutMax=[]  IntegratorOutMin=[]  IntegratorOutMax=[]  FilterOutMin=[]  FilterOutMax=[]  SumOutMin=[]  SumOutMax=[]  SumI1OutMin=[]  SumI1OutMax=[]  SumI2OutMin=[]  SumI2OutMax=[]  SumI3OutMin=[]  SumI3OutMax=[]  SumDOutMin=[]  SumDOutMax=[]  SaturationOutMin=[]  SaturationOutMax=[]  IntegratorContinuousStateAttributes=''  IntegratorStateMustResolveToSignalObject=off  IntegratorRTWStateStorageClass=Auto  FilterContinuousStateAttributes=''  FilterStateMustResolveToSignalObject=off  FilterRTWStateStorageClass=Auto  DifferentiatorICPrevScaledInput=0  DifferentiatorOutMin=[]  DifferentiatorOutMax=[]  FilterDiffOutCoefMin=[]  FilterDiffOutCoefMax=[]  SumDenOutMin=[]  SumDenOutMax=[]  SumNumOutMin=[]  SumNumOutMax=[]  ReciprocalOutMin=[]  ReciprocalOutMax=[]  DivideOutMin=[]  DivideOutMax=[]  TunerSelectOption=Transfer Function Based (PID Tuner App)
  Display{,1..3} (4 alike) : Display
  If : If  IfExpression=u1 > 1
  If Action Subsystem : Subsystem  TreatAsAtomicUnit=on
  If Action Subsystem1 : Subsystem  TreatAsAtomicUnit=on
  Memory : Memory
  Merge : Merge
  Mux1 : Mux  Inputs=2
  Normalization2 : Gain  Gain=1/300
  Saturation : Saturate  UpperLimit=1  LowerLimit=-1
  links : Constant  Value=140
  theta_d1 : Constant  Value=0
  steering angle : Outport  InitialOutput=[0]
  Output : Outport  Port=2
  wires:
  Saturation/1 -> steering angle/1  "Auto steering"
  Memory/1 -> If/1, Display/1, Add/2
  Demux1/2 -> Discrete PID Controller/1
  links/1 -> Mux1/2
  Mux1/1 -> Add1/2  "desired values"
  theta_d1/1 -> Mux1/1
  Add/1 -> Memory/1
  Demux1/1 -> Discrete PID Controller1/1
  Discrete PID Controller/1 -> Display2/1, Add3/2
  In2/1 -> Add1/1
  Normalization2/1 -> Saturation/1
  Constant2/1 -> Add/1
  Add1/1 -> Display3/1, Demux1/1  "Lane error"
  Discrete PID Controller1/1 -> Display1/1, Add3/1
  Add3/1 -> Normalization2/1  "Steering angle"
  If/2 -> If Action Subsystem1/Action
  Merge/1 -> Output/1
  Constant6/1 -> If Action Subsystem1/1(In1)
  If Action Subsystem1/1(Out1) -> Merge/2
  If Action Subsystem/1(Out1) -> Merge/1
  If/1 -> If Action Subsystem/Action
  Constant5/1 -> If Action Subsystem/1(In1)

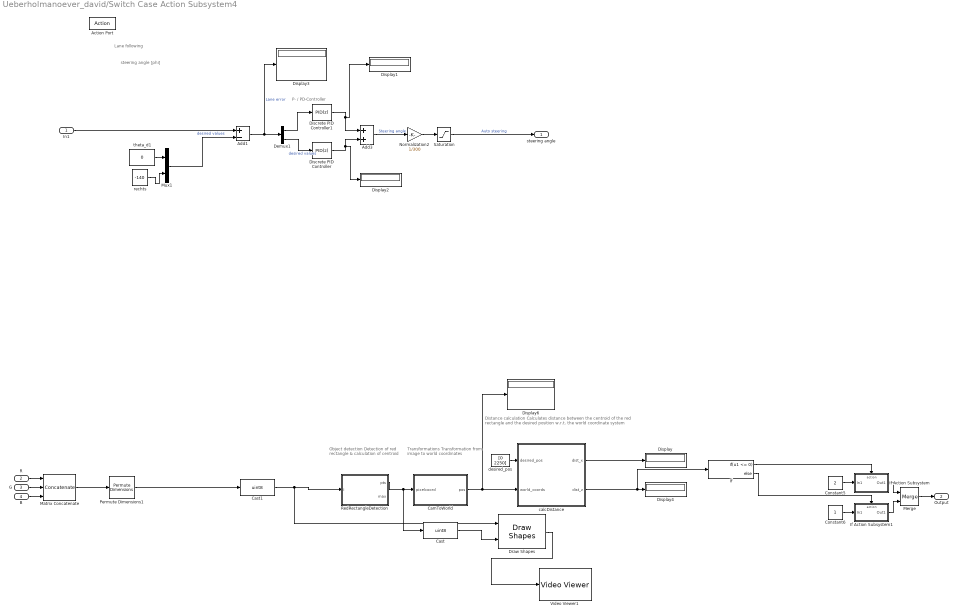
== system Ueberholmanoever_david/Switch Case Action Subsystem4 ==
  note: steering angle [phi]
  note: Transformations
      |
      | Transformation from image
      | to world coordinates
  note: Object detection
      |
      | Detection of red rectangle &
      | calculation of centroid
  note: Lane following
  note: Distance calculation
      |
      | Calculates distance between the centroid of the red rectangle
      | and the desired position w.r.t. the world coordinate system
  note: P- / PD-Controller
  In1 : Inport
  R : Inport  Port=2
  G : Inport  Port=3
  B : Inport  Port=4
  Action Port : ActionPort  ActionType=case
  Add1 : Sum  Inputs=+-
  Add3 : Sum
  CamToWorld : MATLAB Function  TreatAsAtomicUnit=on
  Cast : DataTypeConversion  OutDataTypeStr=uint8
  Cast1 : DataTypeConversion  OutDataTypeStr=uint8
  Constant5 : Constant  Value=2  OutDataTypeStr=uint8
  Constant6 : Constant  OutDataTypeStr=uint8
  Demux1 : Demux  Outputs=2
  Discrete PID Controller : simulink/Continuous/PID Controller  Controller=PID  TimeDomain=Discrete-time  SampleTime=-1  IntegratorMethod=Forward Euler  FilterMethod=Forward Euler  Form=Parallel  UseFilter=on  ControllerParametersSource=internal  P=0.2  I=0  D=0  N=100  InitialConditionSource=internal  InitialConditionForIntegrator=0  InitialConditionForFilter=0  ExternalReset=none  LimitOutput=off  UpperSaturationLimit=inf  LowerSaturationLimit=-inf  LinearizeAsGain=off  AntiWindupMode=none  Kb=1  TrackingMode=off  Kt=1  PParamMin=[]  PParamMax=[]  IParamMin=[]  IParamMax=[]  DParamMin=[]  DParamMax=[]  NParamMin=[]  NParamMax=[]  KbParamMin=[]  KbParamMax=[]  KtParamMin=[]  KtParamMax=[]  POutMin=[]  POutMax=[]  IOutMin=[]  IOutMax=[]  DOutMin=[]  DOutMax=[]  NOutMin=[]  NOutMax=[]  KbOutMin=[]  KbOutMax=[]  KtOutMin=[]  KtOutMax=[]  IntegratorOutMin=[]  IntegratorOutMax=[]  FilterOutMin=[]  FilterOutMax=[]  SumOutMin=[]  SumOutMax=[]  SumI1OutMin=[]  SumI1OutMax=[]  SumI2OutMin=[]  SumI2OutMax=[]  SumI3OutMin=[]  SumI3OutMax=[]  SumDOutMin=[]  SumDOutMax=[]  SaturationOutMin=[]  SaturationOutMax=[]  IntegratorContinuousStateAttributes=''  IntegratorStateMustResolveToSignalObject=off  IntegratorRTWStateStorageClass=Auto  FilterContinuousStateAttributes=''  FilterStateMustResolveToSignalObject=off  FilterRTWStateStorageClass=Auto  DifferentiatorICPrevScaledInput=0  DifferentiatorOutMin=[]  DifferentiatorOutMax=[]  FilterDiffOutCoefMin=[]  FilterDiffOutCoefMax=[]  SumDenOutMin=[]  SumDenOutMax=[]  SumNumOutMin=[]  SumNumOutMax=[]  ReciprocalOutMin=[]  ReciprocalOutMax=[]  DivideOutMin=[]  DivideOutMax=[]  TunerSelectOption=Transfer Function Based (PID Tuner App)
  Discrete PID Controller1 : simulink/Continuous/PID Controller  Controller=PID  TimeDomain=Discrete-time  SampleTime=-1  IntegratorMethod=Forward Euler  FilterMethod=Forward Euler  Form=Parallel  UseFilter=on  ControllerParametersSource=internal  P=6  I=0  D=0  N=100  InitialConditionSource=internal  InitialConditionForIntegrator=0  InitialConditionForFilter=0  ExternalReset=none  LimitOutput=off  UpperSaturationLimit=inf  LowerSaturationLimit=-inf  LinearizeAsGain=off  AntiWindupMode=none  Kb=1  TrackingMode=off  Kt=1  PParamMin=[]  PParamMax=[]  IParamMin=[]  IParamMax=[]  DParamMin=[]  DParamMax=[]  NParamMin=[]  NParamMax=[]  KbParamMin=[]  KbParamMax=[]  KtParamMin=[]  KtParamMax=[]  POutMin=[]  POutMax=[]  IOutMin=[]  IOutMax=[]  DOutMin=[]  DOutMax=[]  NOutMin=[]  NOutMax=[]  KbOutMin=[]  KbOutMax=[]  KtOutMin=[]  KtOutMax=[]  IntegratorOutMin=[]  IntegratorOutMax=[]  FilterOutMin=[]  FilterOutMax=[]  SumOutMin=[]  SumOutMax=[]  SumI1OutMin=[]  SumI1OutMax=[]  SumI2OutMin=[]  SumI2OutMax=[]  SumI3OutMin=[]  SumI3OutMax=[]  SumDOutMin=[]  SumDOutMax=[]  SaturationOutMin=[]  SaturationOutMax=[]  IntegratorContinuousStateAttributes=''  IntegratorStateMustResolveToSignalObject=off  IntegratorRTWStateStorageClass=Auto  FilterContinuousStateAttributes=''  FilterStateMustResolveToSignalObject=off  FilterRTWStateStorageClass=Auto  DifferentiatorICPrevScaledInput=0  DifferentiatorOutMin=[]  DifferentiatorOutMax=[]  FilterDiffOutCoefMin=[]  FilterDiffOutCoefMax=[]  SumDenOutMin=[]  SumDenOutMax=[]  SumNumOutMin=[]  SumNumOutMax=[]  ReciprocalOutMin=[]  ReciprocalOutMax=[]  DivideOutMin=[]  DivideOutMax=[]  TunerSelectOption=Transfer Function Based (PID Tuner App)
  Display{,1..4,6} (6 alike) : Display
  Draw Shapes : visiontextngfix/Draw Shapes  shape=Circles  fill=off  lineWidth=1  fillClrSource=Specify via dialog  display=User-specified value  intensity=200  color=[0 0 255]  opacity=0.6  viewport=Entire image  antialiasing=on  inType=Obsolete  imagePorts=One multidimensional signal  prodOutputMode=Binary point scaling  prodOutputWordLength=32  prodOutputFracLength=14  memoryMode=Specify word length  memoryWordLength=16  memoryFracLength=14  roundingMode=Floor  overflowMode=off
      settings: SourceProductName=Computer Vision System Toolbox
  If : If  IfExpression=u1 <= 0
  If Action Subsystem : Subsystem  TreatAsAtomicUnit=on
  If Action Subsystem1 : Subsystem  TreatAsAtomicUnit=on
  Matrix Concatenate : Concatenate  NumInputs=3  Mode=Multidimensional array  ConcatenateDimension=3
  Merge : Merge
  Mux1 : Mux  Inputs=2
  Normalization2 : Gain  Gain=1/300
  Permute Dimensions1 : PermuteDimensions  Order=[2,1,3]
  RedRectangleDetection : MATLAB Function  TreatAsAtomicUnit=on
  Saturation : Saturate  UpperLimit=1  LowerLimit=-1
  Video Viewer1 : VideoViewer  colormapValue=gray(256)  FigPos=[78 713 770 570]
  "calcDistance " : MATLAB Function  TreatAsAtomicUnit=on
  desired_pos : Constant  Value=[0 2250]
  rechts : Constant  Value=-140
  theta_d1 : Constant  Value=0
  steering angle : Outport  InitialOutput=[0]
  Output : Outport  Port=2
  wires:
  Cast/1 -> Draw Shapes/2
  Matrix Concatenate/1 -> Permute Dimensions1/1
  "calcDistance "/1(dist_x) -> Display/1
  desired_pos/1 -> "calcDistance "/1(desired_pos)
  RedRectangleDetection/1(pts) -> Cast/1, CamToWorld/1(pixelcoord)
  R/1 -> Matrix Concatenate/1
  Permute Dimensions1/1 -> Cast1/1
  Draw Shapes/1 -> Video Viewer1/1
  Demux1/2 -> Discrete PID Controller/1  "desired values"
  If/1 -> If Action Subsystem/Action
  rechts/1 -> Mux1/2
  Constant5/1 -> If Action Subsystem/1(In1)
  Discrete PID Controller/1 -> Display2/1, Add3/2
  Saturation/1 -> steering angle/1  "Auto steering"
  In1/1 -> Add1/1
  Add3/1 -> Normalization2/1  "Steering angle"
  If Action Subsystem/1(Out1) -> Merge/1
  Add1/1 -> Display3/1, Demux1/1  "Lane error"
  Normalization2/1 -> Saturation/1
  Discrete PID Controller1/1 -> Display1/1, Add3/1
  theta_d1/1 -> Mux1/1
  B/1 -> Matrix Concatenate/3
  Cast1/1 -> Draw Shapes/1, RedRectangleDetection/1(I)
  Demux1/1 -> Discrete PID Controller1/1
  G/1 -> Matrix Concatenate/2
  CamToWorld/1(pos) -> "calcDistance "/2(world_coords), Display6/1
  Mux1/1 -> Add1/2  "desired values"
  If/2 -> If Action Subsystem1/Action
  Constant6/1 -> If Action Subsystem1/1(In1)
  If Action Subsystem1/1(Out1) -> Merge/2
  Merge/1 -> Output/1
  "calcDistance "/2(dist_z) -> If/1, Display4/1

== system Ueberholmanoever_david/Switch Case Action Subsystem5 ==
  Video Viewer1 : VideoViewer  colormapValue=gray(256)  FigPos=[78 713 770 570]

== system Ueberholmanoever_david/Switch Case Action Subsystem1/If Action Subsystem ==
  In1 : Inport
  Action Port : ActionPort  ActionType=then
  Out1 : Outport
  wires:
  In1/1 -> Out1/1

== system Ueberholmanoever_david/Switch Case Action Subsystem1/If Action Subsystem1 ==
  In1 : Inport
  Action Port : ActionPort  ActionType=else
  Out1 : Outport
  wires:
  In1/1 -> Out1/1

== system Ueberholmanoever_david/Switch Case Action Subsystem2/If Action Subsystem ==
  In1 : Inport
  Action Port : ActionPort  ActionType=then
  Out1 : Outport
  wires:
  In1/1 -> Out1/1

== system Ueberholmanoever_david/Switch Case Action Subsystem2/If Action Subsystem1 ==
  In1 : Inport
  Action Port : ActionPort  ActionType=else
  Out1 : Outport
  wires:
  In1/1 -> Out1/1

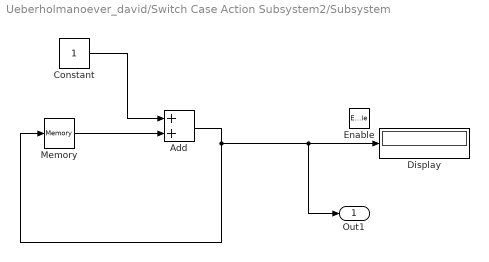
== system Ueberholmanoever_david/Switch Case Action Subsystem2/Subsystem ==
  Enable : EnablePort
  Add : Sum
  Constant : Constant
  Display : Display
  Memory : Memory
  Out1 : Outport  InitialOutput=[0]
  wires:
  Add/1 -> Memory/1, Out1/1, Display/1
  Memory/1 -> Add/2
  Constant/1 -> Add/1

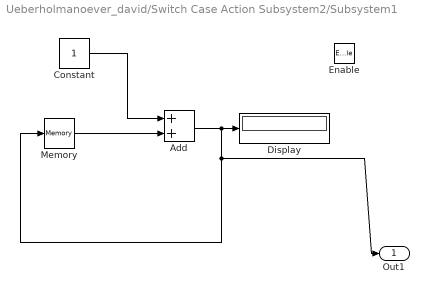
== system Ueberholmanoever_david/Switch Case Action Subsystem2/Subsystem1 ==
  Enable : EnablePort  StatesWhenEnabling=reset  PropagateVarSize=During execution
  Add : Sum
  Constant : Constant
  Display : Display
  Memory : Memory
  Out1 : Outport  OutputWhenDisabled=reset  InitialOutput=[0]
  wires:
  Add/1 -> Out1/1, Memory/1, Display/1
  Memory/1 -> Add/2
  Constant/1 -> Add/1

== system Ueberholmanoever_david/Switch Case Action Subsystem3/If Action Subsystem ==
  In1 : Inport
  Action Port : ActionPort  ActionType=then
  Out1 : Outport
  wires:
  In1/1 -> Out1/1

== system Ueberholmanoever_david/Switch Case Action Subsystem3/If Action Subsystem1 ==
  In1 : Inport
  Action Port : ActionPort  ActionType=else
  Out1 : Outport
  wires:
  In1/1 -> Out1/1

== system Ueberholmanoever_david/Switch Case Action Subsystem4/If Action Subsystem ==
  In1 : Inport
  Action Port : ActionPort  ActionType=then
  Out1 : Outport
  wires:
  In1/1 -> Out1/1

== system Ueberholmanoever_david/Switch Case Action Subsystem4/If Action Subsystem1 ==
  In1 : Inport
  Action Port : ActionPort  ActionType=else
  Out1 : Outport
  wires:
  In1/1 -> Out1/1

== matlab function Ueberholmanoever_david/Lane-finding/Calculate angle ==
  data: lines input; angle output; Pts output; Pts_d output; Ref_I input
function [angle, Pts, Pts_d] = angle(lines, Ref_I)

IMAGE_SIZE = size(Ref_I);
IMAGE_HEIGHT = IMAGE_SIZE(1);
IMAGE_WIDTH = IMAGE_SIZE(2);
points = zeros(2,4);

% Sorting the lines
if double(lines(1,1)) < double(lines(2,1))
    points(1,:) = lines(1,:);
    points(2,:) = lines(2,:);
else
    points(1,:) = lines(2,:);
    points(2,:) = lines(1,:);
end

% Calculate the lane center, top and bottom
x_center = double((points(1,:) + points(2,:))/2);

% Calculate the angle of the centerline: 0 -> vertical
angle = atan((x_center(3) - x_center(1))/IMAGE_HEIGHT);

% Auxilliary lines
Pts = int32([x_center(1), 1, x_center(3), 75]);
Pts_d = int32([IMAGE_WIDTH/2, 1, IMAGE_WIDTH/2, 75]);

% angles = atan2d(double((lines(:,1) - lines(:,3))), -double(lines(:,2) - lines(:,4)));

== matlab function Ueberholmanoever_david/Lane-finding/Calculate center line ==
  data: center_line output; line_center output; lines input; Ref_I input
function [center_line, line_center] = center(lines, Ref_I)

IMAGE_SIZE = size(Ref_I);
IMAGE_HEIGHT = IMAGE_SIZE(1);
IMAGE_WIDTH = IMAGE_SIZE(2);
points = zeros(2,4);

% Sorting the lines
if double(lines(1,1)) < double(lines(2,1))
    points(1,:) = lines(1,:);
    points(2,:) = lines(2,:);
else
    points(1,:) = lines(2,:);
    points(2,:) = lines(1,:);
end

% Calculate the lane center, top and bottom
x_center = double((points(1,:) + points(2,:))/2);

% Output the lane center at the bottom of the picture
line_center = x_center(3);
center_line = x_center;
